simulink model "singlephasedualconverter"  (R2018a)
settings: Solver=VariableStepAuto  StartTime=0.0  StopTime=0.08  RelTol=1e-4
libraries: powerlib x22
settings Model: Creator=chron  LastModifiedBy=chron

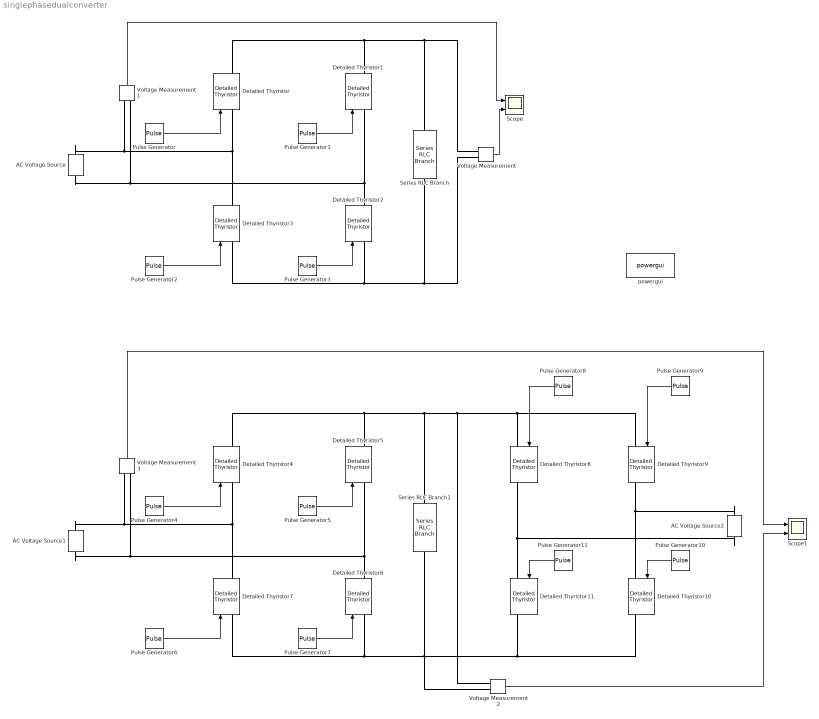
== system singlephasedualconverter ==
  AC Voltage Source : powerlib/Electrical Sources/AC Voltage Source  Amplitude=230  Phase=0  Frequency=50  SampleTime=0  Measurements=None  BusType=swing  Pref=10e3  Qref=0  Qmin=-inf  Qmax=+inf
  AC Voltage Source1 : powerlib/Electrical Sources/AC Voltage Source  Amplitude=230  Phase=0  Frequency=50  SampleTime=0  Measurements=None  BusType=swing  Pref=10e3  Qref=0  Qmin=-inf  Qmax=+inf
  AC Voltage Source2 : powerlib/Electrical Sources/AC Voltage Source  Amplitude=230  Phase=0  Frequency=50  SampleTime=0  Measurements=None  BusType=swing  Pref=10e3  Qref=0  Qmin=-inf  Qmax=+inf
  Detailed Thyristor{,1..11} (12 alike) : powerlib/Power Electronics/Detailed Thyristor  Ron=0.001  Lon=1e-3  Vf=0.8  IL=0.1  Tq=100e-6  IC=0  Rs=500  Cs=250e-9  Measurements=on
      settings: SourceProductName=Simscape Power Systems  SourceProductBaseCode=PS
  Pulse Generator : DiscretePulseGenerator  PulseType=Time based  Period=.02  PulseWidth=5  PhaseDelay=30/360*0.02
  Pulse Generator{1..2,5..6} (4 alike) : DiscretePulseGenerator  PulseType=Time based  Period=0.02  PulseWidth=5  PhaseDelay=210/360*0.02
  Pulse Generator10 : DiscretePulseGenerator  PulseType=Time based  Period=0.02  PulseWidth=5  PhaseDelay=150/360*0.02
  Pulse Generator11 : DiscretePulseGenerator  PulseType=Time based  Period=0.02  PulseWidth=5  PhaseDelay=330/360*0.02
  Pulse Generator3 : DiscretePulseGenerator  PulseType=Time based  Period=0.02  PulseWidth=5  PhaseDelay=30/360*0.02
  Pulse Generator4 : DiscretePulseGenerator  PulseType=Time based  Period=.02  PulseWidth=5  PhaseDelay=30/360*0.02
  Pulse Generator7 : DiscretePulseGenerator  PulseType=Time based  Period=0.02  PulseWidth=5  PhaseDelay=30/360*0.02
  Pulse Generator8 : DiscretePulseGenerator  PulseType=Time based  Period=0.02  PulseWidth=5  PhaseDelay=150/360*0.02
  Pulse Generator9 : DiscretePulseGenerator  PulseType=Time based  Period=0.02  PulseWidth=5  PhaseDelay=330/360*0.02
  Scope : Scope  NumInputPorts=2
  Scope1 : Scope  NumInputPorts=2
  Series RLC Branch : powerlib/Elements/Series RLC Branch  LConnTagsString=__new0  RConnTagsString=__new0  BranchType=R  Resistance=10e-4  Inductance=1e-3  SetiL0=off  InitialCurrent=0  Capacitance=1e-6  Setx0=off  InitialVoltage=0  Measurements=None
  Series RLC Branch1 : powerlib/Elements/Series RLC Branch  LConnTagsString=__new0  RConnTagsString=__new0  BranchType=R  Resistance=10  Inductance=1e-3  SetiL0=off  InitialCurrent=0  Capacitance=1e-6  Setx0=off  InitialVoltage=0  Measurements=None
  Voltage Measurement{,1..3} (4 alike) : powerlib/Measurements/Voltage Measurement  PhasorSimulation=off  OutputType=Complex  PSBequivalent=0
  powergui : powerlib/powergui  Priority=1  SimulationMode=Continuous  SampleTime=50e-6  frequency=60  Iterations=50  frequencyindice=0  Pbase=100e6  ErrMax=1e-4  UnitsV=kV  UnitsW=MW  buscounter=0  FunctionMessages=off  echomessages=off  EnableUseOfTLC=off  CurrentSourceSwitches=off  DisableSnubberDevices=off  DisableRonSwitches=off  DisableVfSwitches=off  DisplayEquations=off  SolverType=Tustin/Backward Euler (TBE)  Interpol=off  ExternalGateDelay=off  methode=off  Ts=100  x0status=blocks  SPID=on  SwTol=0  HookPort=off  RestoreLinks=warning  ResistiveCurrentMeasurement=off  Frange=[0:2:500]  Ylog=off  Xlog=on  ShowGrid=off  save=off  variable=ZData  structure=0  ZoomFFT=off  StartTime=0.0  cycles=1  DisplayStyle=1  fundamental=60  FreqAxis=off  MaxFrequency=1000  frequencyindicesteady=1  RmsSteady=1  display=off
  wires:
  Pulse Generator/1 -> Detailed Thyristor/1
  Pulse Generator1/1 -> Detailed Thyristor1/1
  Pulse Generator3/1 -> Detailed Thyristor2/1
  Pulse Generator2/1 -> Detailed Thyristor3/1
  Voltage Measurement/1 -> Scope/2
  Voltage Measurement1/1 -> Scope/1
  Voltage Measurement3/1 -> Scope1/1
  Voltage Measurement2/1 -> Scope1/2
  Pulse Generator6/1 -> Detailed Thyristor7/1
  Pulse Generator4/1 -> Detailed Thyristor4/1
  Pulse Generator7/1 -> Detailed Thyristor6/1
  Pulse Generator5/1 -> Detailed Thyristor5/1
  Pulse Generator10/1 -> Detailed Thyristor10/1
  Pulse Generator9/1 -> Detailed Thyristor9/1
  Pulse Generator8/1 -> Detailed Thyristor8/1
  Pulse Generator11/1 -> Detailed Thyristor11/1
  connections:
  Detailed Thyristor/RConn1 -- Voltage Measurement/LConn1 -- Series RLC Branch/RConn1 -- Detailed Thyristor1/RConn1
  Detailed Thyristor2/RConn1 -- AC Voltage Source/LConn1 -- Voltage Measurement1/LConn2 -- Detailed Thyristor1/LConn1
  Detailed Thyristor2/LConn1 -- Voltage Measurement/LConn2 -- Series RLC Branch/LConn1 -- Detailed Thyristor3/LConn1
  Detailed Thyristor/LConn1 -- AC Voltage Source/RConn1 -- Voltage Measurement1/LConn1 -- Detailed Thyristor3/RConn1
  Detailed Thyristor4/RConn1 -- Series RLC Branch1/LConn1 -- Detailed Thyristor8/LConn1 -- Detailed Thyristor9/LConn1 -- Voltage Measurement2/LConn1 -- Detailed Thyristor5/RConn1
  Detailed Thyristor7/LConn1 -- Detailed Thyristor6/LConn1 -- Series RLC Branch1/RConn1 -- Detailed Thyristor11/RConn1 -- Detailed Thyristor10/RConn1 -- Voltage Measurement2/LConn2
  Detailed Thyristor7/RConn1 -- Detailed Thyristor4/LConn1 -- AC Voltage Source1/RConn1 -- Voltage Measurement3/LConn1
  Detailed Thyristor5/LConn1 -- Detailed Thyristor6/RConn1 -- AC Voltage Source1/LConn1 -- Voltage Measurement3/LConn2
  Detailed Thyristor8/RConn1 -- AC Voltage Source2/LConn1 -- Detailed Thyristor11/LConn1
  Detailed Thyristor9/RConn1 -- AC Voltage Source2/RConn1 -- Detailed Thyristor10/LConn1
